simulink model "Fig279"  (R2014b)
settings: Solver=ode3  StartTime=0.0  StopTime=24.576  FixedStep=1e-4  RelTol=1e-5
libraries: commrandsrc2 x1
settings Model: Creator=Dennis Silage  LastModifiedBy=Silage
settings DataIOCC: SignalLoggingSaveFormat=ModelDataLogs
settings OptimizationCC: ExpressionDepthLimit=2147483647  InitFltsAndDblsToZero=on
settings DebuggingCC: UnderspecifiedInitializationDetection=Classic  MergeDetectMultiDrivingBlocksExec=none  SolverPrmCheckMsg=none  FcnCallInpInsideContextMsg=UseLocalSettings  StateNameClashWarn=warning
settings GRTTargetCC: CombineOutputUpdateFcns=off  GRTInterface=on

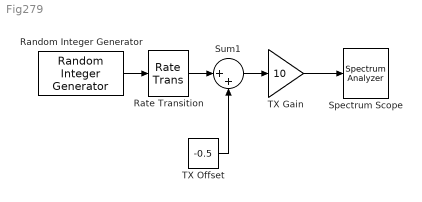
== system Fig279 ==
  Random Integer Generator : commrandsrc2/Random Integer Generator  mul=2  seed=randseed  Ts=1e-3  frameBased=off  sampPerFrame=50  orient=on  outDataType=double
  Rate Transition : RateTransition  OutPortSampleTime=1e-4
  Spectrum Scope : SpectrumAnalyzer
  Sum1 : Sum  Inputs=|++
  TX Gain : Gain  Gain=10
  TX Offset : Constant  Value=-0.5
  wires:
  Random Integer Generator/1 -> Rate Transition/1
  Rate Transition/1 -> Sum1/1
  Sum1/1 -> TX Gain/1
  TX Offset/1 -> Sum1/2
  TX Gain/1 -> Spectrum Scope/1
